simulink model "channelizer_FIR1"  (R2025a)
settings: Solver=VariableStepAuto  StartTime=0.0  StopTime=4000/100e6  RelTol=1e-3
InitFcn:
  | num_chan = 8;  % Number of channels
  | taps_per_phase = 20; % Number of taps per channel.
  | count = 1;
  | for i=0:1:num_chan-1 % number of channels
  |       coeffs_set_num(count:count+taps_per_phase+2) = i;
  |       count = count + taps_per_phase+2;
  |      if i == 0
  |        coeffs_set_num(count:count+5) = 0;
  |        count = count + 5;
  |      else
  |        coeffs_set_num(count:count+2) = 0;
  |        count = count + 2;
  |     end
  | 
  | end
  | 
  | coeffs_set_num = coeffs_set_num(1:160);
  | coeffs_tlast = [zeros(1,num_chan)];
  | for k=1:1:39
  | coeffs_tlast = [coeffs_tlast,1,zeros(1,(num_chan/2)-1)];
  | end
  | coeffs_tlast = coeffs_tlast(1:160);
undefined symbols (not defined in the file or in its folder): dspblkCoreblockFVToolHelper, es1, gcbh, S, vsva2488, xcvr1602
libraries: hdlBasic x30, dspsrcs4 x4, dspswit3 x2, hdlDSPIP x1, vmcUtilities x1
settings Model: Creator=nanumolu  LastModifiedBy=sdegala

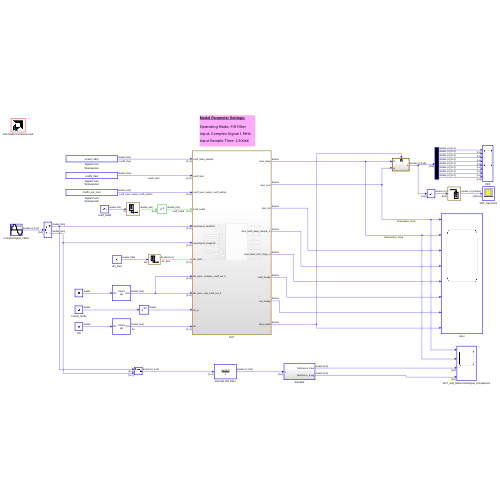
[thumbnail: Simulink's stored preview of the top-level diagram]
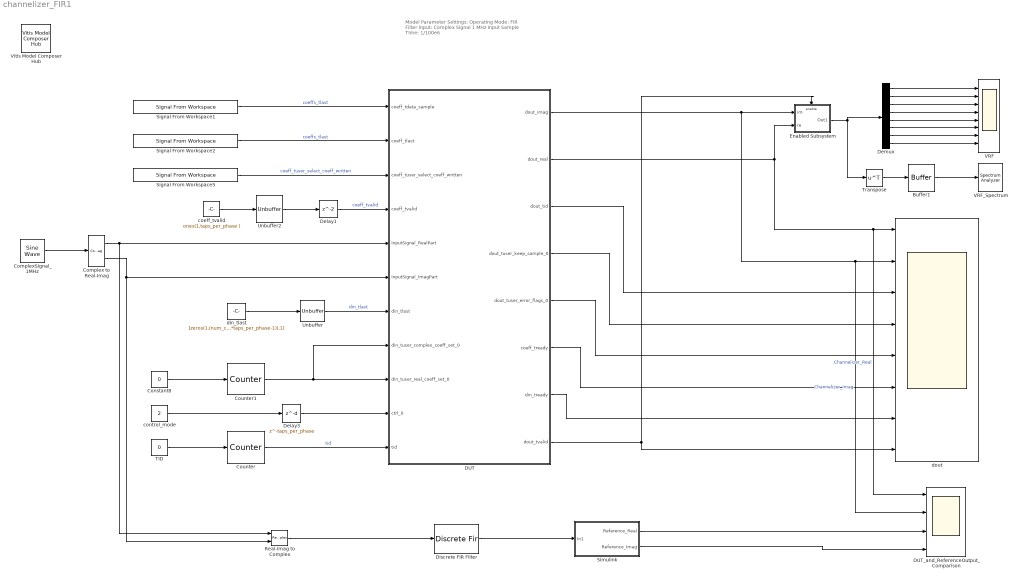
== system channelizer_FIR1 ==
  note: Model Parameter Settings:
      |
      | Operating Mode: FIR Filter
      | Input: Complex Signal 1 MHz
      | Input Sample TIme: 1/100e6
  Buffer1 : Buffer  N=1024  OutputFrames=off
  Complex to Real-Imag : ComplexToRealImag
  ComplexSignal_1MHz : dspsrcs4/Sine Wave  Amplitude=0.15  Frequency=1e6  Phase=0  SampleMode=Discrete  OutComplex=Complex  CompMethod=Trigonometric fcn  TableSize=Speed  SampleTime=1/100e6  SamplesPerFrame=1  ResetState=Restart at time zero  OutputFrames=off  dataType=double  wordLen=16  udDataType=sfix(16)  fracBitsMode=Best precision  numFracBits=15  OutDataTypeStr=double  LastOutDataTypeStr=double
  Constant8 : Constant  Value=0  SampleTime=1/100e6
  Counter : dspswit3/Counter  Direction=Up  CountEvent=Non-zero sample  CounterSize=User defined  MaxCount=num_chan-1  InitialCount=0  Output=Count  HitValue=32  ResetInput=off  SamplesPerFrame=1  Ts=1  CntDtype=double  HitDtype=Logical
  Counter1 : dspswit3/Counter  Direction=Up  CountEvent=Non-zero sample  CounterSize=User defined  MaxCount=num_chan-1  InitialCount=0  Output=Count  HitValue=32  ResetInput=off  SamplesPerFrame=1  Ts=1  CntDtype=double  HitDtype=Logical
  DUT : Subsystem
  DUT_and_ReferenceOutput_Comparison : Scope  NumInputPorts=4
      settings: ActiveDisplayYMinimum=-0.44039726257324219  ActiveDisplayYMaximum=0.44039726257324219
  Delay1 : Delay
  Delay3 : Delay  DelayLength=taps_per_phase
  Demux : Demux  Outputs=8
  Discrete FIR Filter : DiscreteFir  LoadFcn=dspblkCoreblockFVToolHelper(gcbh,'load');  Coefficients=ones(1,20)  InputProcessing=Columns as channels (frame based)  OutDataTypeStr=Inherit: Same as input
      settings: CopyFcn=dspblkCoreblockFVToolHelper(gcbh,'copy');  DeleteFcn=dspblkCoreblockFVToolHelper(gcbh,'close');  ModelCloseFcn=dspblkCoreblockFVToolHelper(gcbh,'close');  PreSaveFcn=dspblkCoreblockFVToolHelper(gcbh,'presave');  PostSaveFcn=dspblkCoreblockFVToolHelper(gcbh,'postsave');  CloseFcn=dspblkCoreblockFVToolHelper(gcbh,'close');
  Enabled Subsystem : Subsystem  TreatAsAtomicUnit=on
  Real-Imag to Complex : RealImagToComplex
  Signal From Workspace1 : dspsrcs4/Signal From Workspace  X=ones(1,160)  Ts=1/100e6  nsamps=1  OutputAfterFinalValue=Setting to zero  ignoreOrWarnInputAndFrameLengths=off  OutputFrames=off
  Signal From Workspace2 : dspsrcs4/Signal From Workspace  X=coeffs_tlast  Ts=1/100e6  nsamps=1  OutputAfterFinalValue=Setting to zero  ignoreOrWarnInputAndFrameLengths=off  OutputFrames=off
  Signal From Workspace5 : dspsrcs4/Signal From Workspace  X=coeffs_set_num  Ts=1/100e6  nsamps=1  OutputAfterFinalValue=Setting to zero  ignoreOrWarnInputAndFrameLengths=off  OutputFrames=off
  Simulink : Subsystem
  TID : Constant  Value=0  SampleTime=1
  Transpose : Math  Operator=transpose
  Unbuffer : Unbuffer
  Unbuffer2 : Unbuffer
  VRF : Scope  NumInputPorts=8
      settings: TimeUnits=Metric (based on Time Span)  ActiveDisplayYMinimum=-0.43884372711181641  ActiveDisplayYMaximum=0.44022464752197266  YLabel=Amplitude  DataLoggingVariableName=ScopeData3
  VRF_Spectrum : SpectrumAnalyzer  WindowPosition=[1.000000,1.000000,1920.000000,1127.000000,]  Visible=on  ScopeFrameLocation=window  WindowInvariantSamplesPerUpdate=on  Span=100000000  StartFrequency=-50000000  StopFrequency=50000000  YLimits=[-3603.4449 -2802.6794]
  Vitis Model Composer Hub : vmcUtilities/Vitis Model Composer Hub  Tag=genX  CodeGeneration=off  SubsystemName=DUT  BlockHierPath=Channalizer_smoke  CompilationType=HDLCompilation  SubsystemType=HDLNode  ExportTypeV2=HDL Netlist  StartColumn=1  NumberOfColumns=1  TargetDirectory=./netlist_chan_vlg  exportDesign=on  analyzeDesign=off  validateDesignOnHw=off  ExportType=AI Engines  IpVendor=xilinx.com  IpLibrary=hls  IpVersion=1.0  IpHWLanguage=Verilog  AieCompilerOptions={}  AieSimulatorOptions={}  CreateTestbench=on  TestbenchStackSize=10  RunRtlSim=off  RunCSim=off  RunAieSim=off  AieSimTimeout=50000  RunAieSimProfiling=off  LaunchVitisAnalyzer=off  PlotOutput=off  RunX86Sim=off  X86SimTimeout=10  GenHwImage=off  GenLibadfXo=on  GenHwValidationCode=off  PlatformType=Not Specified  HwSystemType=Baremetal  HwValidationTarget=hw  ProjDevice=xcvr1602-vsva2488-2MP-e-S-es1  ProjDevicePart=xcvr1602-vsva2488-2MP-e-S-es1  AIEType=AIE  SamplePeriod=-1  ClockFrequency=200  DataPathParallelism=1  xilinxfamily=versalairfes1  part=xcvr1602  speed=-2MP-e-S-es1  package=vsva2488  directory=./netlist/ip/DUT/src  testbench=off  incr_netlist=off  synthesis_tool=Vivado  clock_wrapper=Clock Enables  dbl_ovrd=According to Block Masks  dcm_input_clock_period=10  sysclk_period=10  simulink_period=1/100e6  eval_field=0  IPInfoJsonString="{\"DUTSubsystemName\":\"Channalizer_smoke\",\"HDLSubsystem\":{\"SubsystemName\":\"Channalizer_smoke\",\"IPName\":\"Copy_of_hamilton_vrf_fft\",\"IPLibrary\":\"VMC\",\"IPVendor\":\"User Company\",\"IPVersion\":\"1.0\",\"TargetDirectory\":\"./netlist_chan_vlg\",\"SubsystemDir\":\"./netlist_chan_vlg/ip/Channalizer_smoke\",\"FreqHz\":\"100000000\"},\"SubsystemTag\":\"HDLNode\"}"  LogFileName=/proj/dsv_xhd/ravalib/Head/Tests/REL/2025.1/dsv/modelcomposer/hdl/regression/channelizer/smoke/netlist_chan_vlg/model_composer.log  NThreads=4  IPConfigFile=/tmp/vmctmp-10364637636032824832/Channalizer_smoke_ipconfig.json
  coeff_tvalid : Constant  Value=ones(1,taps_per_phase )  SampleTime=1/100e6
  control_mode : Constant  Value=2  SampleTime=1/100e6
  din_tlast : Constant  Value=[zeros(1,(num_chan*taps_per_phase-1)),1]  SampleTime=1/100e6
  dout : Scope  NumInputPorts=8
      settings: ActiveDisplayYMinimum=-0.44039726257324219  ActiveDisplayYMaximum=0.44039726257324219
  wires:
  Delay1/1 -> DUT/4(coeff_tvalid)  "coeff_tvalid"
  Unbuffer/1 -> DUT/7(din_tlast)  "din_tlast"
  Counter1/1 -> DUT/8(din_tuser_complex_coeff_set_0), DUT/9(din_tuser_real_coeff_set_0)
  Complex to Real-Imag/2 -> Real-Imag to Complex/2, DUT/6(InputSignal_ImagPart)
  din_tlast/1 -> Unbuffer/1
  TID/1 -> Counter/1
  coeff_tvalid/1 -> Unbuffer2/1
  Unbuffer2/1 -> Delay1/1
  control_mode/1 -> Delay3/1
  Constant8/1 -> Counter1/1
  DUT/2(dout_real) -> Enabled Subsystem/2(re), DUT_and_ReferenceOutput_Comparison/1, dout/1  "Channelizer_Real"
  DUT/1(dout_imag) -> Enabled Subsystem/1(im), dout/2, DUT_and_ReferenceOutput_Comparison/2  "Channelizer_Imag"
  Signal From Workspace5/1 -> DUT/3(coeff_tuser_select_coeff_written)  "coeff_tuser_select_coeff_written"
  DUT/3(dout_tid) -> dout/3
  DUT/4(dout_tuser_keep_sample_0) -> dout/4
  DUT/5(dout_tuser_error_flags_0) -> dout/5
  DUT/6(coeff_tready) -> dout/6
  DUT/7(din_tready) -> dout/7
  Enabled Subsystem/1(Out1) -> Demux/1, Transpose/1
  Buffer1/1 -> VRF_Spectrum/1
  Signal From Workspace2/1 -> DUT/2(coeff_tlast)  "coeffs_tlast"
  Transpose/1 -> Buffer1/1
  Demux/1 -> VRF/1
  Demux/2 -> VRF/2
  Demux/3 -> VRF/3
  Demux/4 -> VRF/4
  Demux/5 -> VRF/5
  Demux/6 -> VRF/6
  Demux/7 -> VRF/7
  Demux/8 -> VRF/8
  Real-Imag to Complex/1 -> Discrete FIR Filter/1
  Delay3/1 -> DUT/10(ctrl_0)
  Counter/1 -> DUT/11(tid)  "tid"
  Complex to Real-Imag/1 -> Real-Imag to Complex/1, DUT/5(InputSignal_RealPart)
  DUT/8(dout_tvalid) -> Enabled Subsystem/Enable, dout/8
  Discrete FIR Filter/1 -> Simulink/1(In1)
  Simulink/1(Reference_Real) -> DUT_and_ReferenceOutput_Comparison/3
  Simulink/2(Reference_Imag) -> DUT_and_ReferenceOutput_Comparison/4
  ComplexSignal_1MHz/1 -> Complex to Real-Imag/1
  Signal From Workspace1/1 -> DUT/1(coeff_tdata_sample)  "coeffs_tlast"

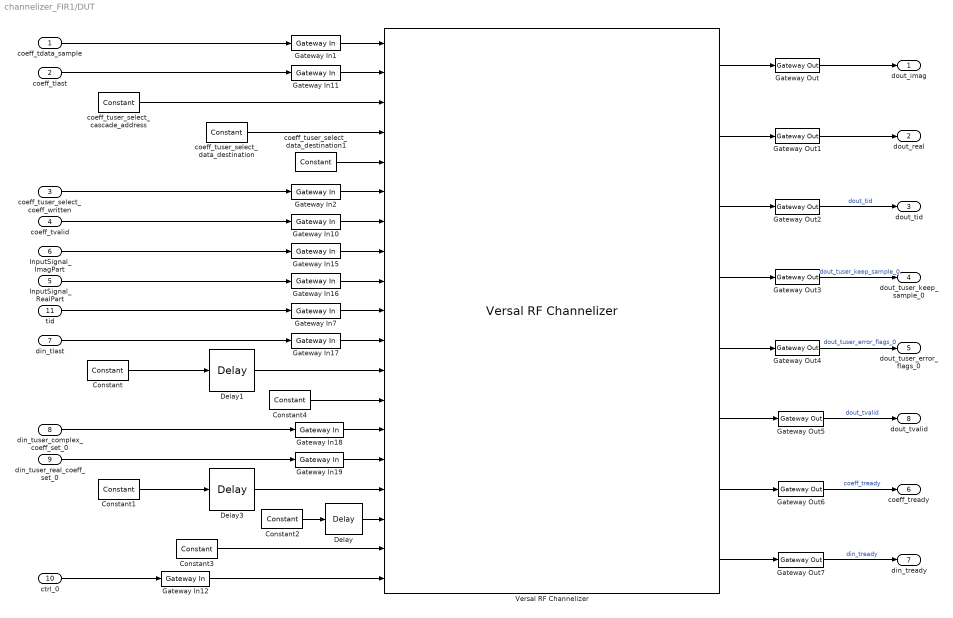
== system channelizer_FIR1/DUT ==
  coeff_tdata_sample : Inport
  coeff_tlast : Inport  Port=2
  coeff_tuser_select_coeff_written : Inport  Port=3
  coeff_tvalid : Inport  Port=4
  InputSignal_RealPart : Inport  Port=5
  InputSignal_ImagPart : Inport  Port=6
  din_tlast : Inport  Port=7
  din_tuser_complex_coeff_set_0 : Inport  Port=8
  din_tuser_real_coeff_set_0 : Inport  Port=9
  ctrl_0 : Inport  Port=10
  tid : Inport  Port=11
  Constant : hdlBasic/Constant  const=1.0  gui_display_data_type=Fixed-point  arith_type=Unsigned  n_bits=1  bin_pt=0  preci_type=Single  exp_width=8  frac_width=24  explicit_period=on  period=1/100e6  XmcBlockStatus=1  maskContainerNames=tabcontainer1  block_type=constant  block_config=sysgen:Constant_config
  Constant1 : hdlBasic/Constant  const=1.0  gui_display_data_type=Boolean  arith_type=Boolean  n_bits=1  bin_pt=0  preci_type=Single  exp_width=8  frac_width=24  explicit_period=on  period=1/100e6  XmcBlockStatus=1  maskContainerNames=tabcontainer1  block_type=constant  block_config=sysgen:Constant_config
  Constant2 : hdlBasic/Constant  const=1.0  gui_display_data_type=Boolean  arith_type=Boolean  n_bits=1  bin_pt=0  preci_type=Single  exp_width=8  frac_width=24  explicit_period=on  period=1/100e6  XmcBlockStatus=1  maskContainerNames=tabcontainer1  block_type=constant  block_config=sysgen:Constant_config
  Constant3 : hdlBasic/Constant  const=1.0  gui_display_data_type=Boolean  arith_type=Boolean  n_bits=1  bin_pt=0  preci_type=Single  exp_width=8  frac_width=24  explicit_period=on  period=1/100e6  XmcBlockStatus=1  maskContainerNames=tabcontainer1  block_type=constant  block_config=sysgen:Constant_config
  Constant4 : hdlBasic/Constant  const=1.0  gui_display_data_type=Fixed-point  arith_type=Unsigned  n_bits=1  bin_pt=0  preci_type=Single  exp_width=8  frac_width=24  explicit_period=on  period=1/100e6  XmcBlockStatus=1  maskContainerNames=tabcontainer1  block_type=constant  block_config=sysgen:Constant_config
  Delay : hdlBasic/Delay  rst=off  en=off  latency=2  reg_retiming=off  XmcBlockStatus=1  maskContainerNames=group1  block_type=delay  block_config=sysgen:Delay_config
  Delay1 : hdlBasic/Delay  rst=off  en=off  latency=num_chan*taps_per_phase  reg_retiming=off  XmcBlockStatus=1  maskContainerNames=group1  block_type=delay  block_config=sysgen:Delay_config
  Delay3 : hdlBasic/Delay  rst=off  en=off  latency=num_chan*taps_per_phase  reg_retiming=off  XmcBlockStatus=1  maskContainerNames=group1  block_type=delay  block_config=sysgen:Delay_config
  Gateway In1 : hdlBasic/Gateway In  gui_display_data_type=Fixed-point  arith_type=Signed (2's comp)  n_bits=18  bin_pt=17  preci_type=Single  exp_width=8  frac_width=24  rows=1  columns=1  quantization="Round  (unbiased: +/- Inf)"  overflow=Saturate  period=1/100e6  UseAsADC=off  ADCChannel='1'  interface=None  automatic_assignment=on  address_offset=hex2dec('00')  intf_name=''  intf_description=''  default_value=0  timing_constraint=None  locs_specified=off  LOCs={}  io_standard={}  inherit_from_input=off  hdl_port=on  XmcBlockStatus=1  maskContainerNames=group4  block_type=gatewayin  block_config=sysgen:gateway_in_config  block_width_w=590  block_height_w=620  block_width=640  block_height=850
  Gateway In10 : hdlBasic/Gateway In  gui_display_data_type=Boolean  arith_type=Boolean  n_bits=16  bin_pt=14  preci_type=Single  exp_width=8  frac_width=24  rows=1  columns=1  quantization="Round  (unbiased: +/- Inf)"  overflow=Saturate  period=1/100e6  UseAsADC=off  ADCChannel='1'  interface=None  automatic_assignment=on  address_offset=hex2dec('00')  intf_name=''  intf_description=''  default_value=0  timing_constraint=None  locs_specified=off  LOCs={}  io_standard={}  inherit_from_input=off  hdl_port=on  XmcBlockStatus=1  maskContainerNames=group4  block_type=gatewayin  block_config=sysgen:gateway_in_config  block_width_w=590  block_height_w=620  block_width=640  block_height=850
  Gateway In11 : hdlBasic/Gateway In  gui_display_data_type=Boolean  arith_type=Boolean  n_bits=16  bin_pt=14  preci_type=Single  exp_width=8  frac_width=24  rows=1  columns=1  quantization="Round  (unbiased: +/- Inf)"  overflow=Saturate  period=1/100e6  UseAsADC=off  ADCChannel='1'  interface=None  automatic_assignment=on  address_offset=hex2dec('00')  intf_name=''  intf_description=''  default_value=0  timing_constraint=None  locs_specified=off  LOCs={}  io_standard={}  inherit_from_input=off  hdl_port=on  XmcBlockStatus=1  maskContainerNames=group4  block_type=gatewayin  block_config=sysgen:gateway_in_config  block_width_w=590  block_height_w=620  block_width=640  block_height=850
  Gateway In12 : hdlBasic/Gateway In  gui_display_data_type=Fixed-point  arith_type=Signed (2's comp)  n_bits=8  bin_pt=0  preci_type=Single  exp_width=8  frac_width=24  rows=1  columns=1  quantization="Round  (unbiased: +/- Inf)"  overflow=Saturate  period=1/100e6  UseAsADC=off  ADCChannel='1'  interface=None  automatic_assignment=on  address_offset=hex2dec('00')  intf_name=''  intf_description=''  default_value=0  timing_constraint=None  locs_specified=off  LOCs={}  io_standard={}  inherit_from_input=off  hdl_port=on  XmcBlockStatus=1  maskContainerNames=group4  block_type=gatewayin  block_config=sysgen:gateway_in_config  block_width_w=590  block_height_w=620  block_width=640  block_height=850
  Gateway In15 : hdlBasic/Gateway In  gui_display_data_type=Fixed-point  arith_type=Signed (2's comp)  n_bits=18  bin_pt=17  preci_type=Single  exp_width=8  frac_width=24  rows=1  columns=1  quantization="Round  (unbiased: +/- Inf)"  overflow=Saturate  period=1/100e6  UseAsADC=off  ADCChannel='1'  interface=None  automatic_assignment=on  address_offset=hex2dec('00')  intf_name=''  intf_description=''  default_value=0  timing_constraint=None  locs_specified=off  LOCs={}  io_standard={}  inherit_from_input=off  hdl_port=on  XmcBlockStatus=1  maskContainerNames=group4  block_type=gatewayin  block_config=sysgen:gateway_in_config  block_width_w=590  block_height_w=620  block_width=640  block_height=850
  Gateway In16 : hdlBasic/Gateway In  gui_display_data_type=Fixed-point  arith_type=Signed (2's comp)  n_bits=18  bin_pt=17  preci_type=Single  exp_width=8  frac_width=24  rows=1  columns=1  quantization="Round  (unbiased: +/- Inf)"  overflow=Saturate  period=1/100e6  UseAsADC=off  ADCChannel='1'  interface=None  automatic_assignment=on  address_offset=hex2dec('00')  intf_name=''  intf_description=''  default_value=0  timing_constraint=None  locs_specified=off  LOCs={}  io_standard={}  inherit_from_input=off  hdl_port=on  XmcBlockStatus=1  maskContainerNames=group4  block_type=gatewayin  block_config=sysgen:gateway_in_config  block_width_w=590  block_height_w=620  block_width=640  block_height=850
  Gateway In17 : hdlBasic/Gateway In  gui_display_data_type=Boolean  arith_type=Boolean  n_bits=16  bin_pt=14  preci_type=Single  exp_width=8  frac_width=24  rows=1  columns=1  quantization="Round  (unbiased: +/- Inf)"  overflow=Saturate  period=1/100e6  UseAsADC=off  ADCChannel='1'  interface=None  automatic_assignment=on  address_offset=hex2dec('00')  intf_name=''  intf_description=''  default_value=0  timing_constraint=None  locs_specified=off  LOCs={}  io_standard={}  inherit_from_input=off  hdl_port=on  XmcBlockStatus=1  maskContainerNames=group4  block_type=gatewayin  block_config=sysgen:gateway_in_config  block_width_w=590  block_height_w=620  block_width=640  block_height=850
  Gateway In18 : hdlBasic/Gateway In  gui_display_data_type=Fixed-point  arith_type=Unsigned  n_bits=3  bin_pt=0  preci_type=Single  exp_width=8  frac_width=24  rows=1  columns=1  quantization="Round  (unbiased: +/- Inf)"  overflow=Saturate  period=1/100e6  UseAsADC=off  ADCChannel='1'  interface=None  automatic_assignment=on  address_offset=hex2dec('00')  intf_name=''  intf_description=''  default_value=0  timing_constraint=None  locs_specified=off  LOCs={}  io_standard={}  inherit_from_input=off  hdl_port=on  XmcBlockStatus=1  maskContainerNames=group4  block_type=gatewayin  block_config=sysgen:gateway_in_config  block_width_w=590  block_height_w=620  block_width=640  block_height=850
  Gateway In19 : hdlBasic/Gateway In  gui_display_data_type=Fixed-point  arith_type=Unsigned  n_bits=3  bin_pt=0  preci_type=Single  exp_width=8  frac_width=24  rows=1  columns=1  quantization="Round  (unbiased: +/- Inf)"  overflow=Saturate  period=1/100e6  UseAsADC=off  ADCChannel='1'  interface=None  automatic_assignment=on  address_offset=hex2dec('00')  intf_name=''  intf_description=''  default_value=0  timing_constraint=None  locs_specified=off  LOCs={}  io_standard={}  inherit_from_input=off  hdl_port=on  XmcBlockStatus=1  maskContainerNames=group4  block_type=gatewayin  block_config=sysgen:gateway_in_config  block_width_w=590  block_height_w=620  block_width=640  block_height=850
  Gateway In2 : hdlBasic/Gateway In  gui_display_data_type=Fixed-point  arith_type=Unsigned  n_bits=3  bin_pt=0  preci_type=Single  exp_width=8  frac_width=24  rows=1  columns=1  quantization="Round  (unbiased: +/- Inf)"  overflow=Saturate  period=1/100e6  UseAsADC=off  ADCChannel='1'  interface=None  automatic_assignment=on  address_offset=hex2dec('00')  intf_name=''  intf_description=''  default_value=0  timing_constraint=None  locs_specified=off  LOCs={}  io_standard={}  inherit_from_input=off  hdl_port=on  XmcBlockStatus=1  maskContainerNames=group4  block_type=gatewayin  block_config=sysgen:gateway_in_config  block_width_w=590  block_height_w=620  block_width=640  block_height=850
  Gateway In7 : hdlBasic/Gateway In  gui_display_data_type=Fixed-point  arith_type=Signed (2's comp)  n_bits=3  bin_pt=0  preci_type=Single  exp_width=8  frac_width=24  rows=1  columns=1  quantization="Round  (unbiased: +/- Inf)"  overflow=Saturate  period=1/100e6  UseAsADC=off  ADCChannel='1'  interface=None  automatic_assignment=on  address_offset=hex2dec('00')  intf_name=''  intf_description=''  default_value=0  timing_constraint=None  locs_specified=off  LOCs={}  io_standard={}  inherit_from_input=off  hdl_port=on  XmcBlockStatus=1  maskContainerNames=group4  block_type=gatewayin  block_config=sysgen:gateway_in_config  block_width_w=590  block_height_w=620  block_width=640  block_height=850
  Gateway Out{,1..7} (8 alike) : hdlBasic/Gateway Out  inherit_from_input=off  bool_to_boolean=off  hdl_port=on  rows=1  columns=1  UseAsDAC=off  DACChannel='1'  interface=None  automatic_assignment=on  address_offset=hex2dec('00')  intf_name=''  intf_description=''  timing_constraint=None  locs_specified=off  LOCs={}  io_standard={}  XmcBlockStatus=1  maskContainerNames=group4  block_type=gatewayout  block_config=sysgen:gateway_out_config  block_width_w=590  block_height_w=620  block_width=620  block_height=750
  Versal RF Channelizer : hdlDSPIP/Versal RF Channelizer  mode=FIR Filter  input_sample_rate=1  num_of_instances=1  fft_direction=FFT  fft_sync_on_tlast=off  fir_coeff_type=Real  fir_length=16  gain_en=off  events=off  coeff_casc_en=off  active_duty_cycle=25  toggle_rate=25  fir_unit_0_taps=16  fir_unit_1_taps=0  fir_unit_2_taps=0  fir_unit_3_taps=0  ip_name=Versal RF Channelizer  enable_all_ports=false  ip_version=1.1  dsptool_ready=false  ipcore_usecache=true  ipcore_useipmodelcache=true  wrapper_available=true  port_translation_map={ 'aclken' => 'en', 'aresetn' => 'rst' }  structural_sim=true  ipcore_do_not_force_period=true  oldconvolution_code_radix=Binary  XmcBlockStatus=1  maskContainerNames=tabcontainer1  block_type=vrf_channelizer_v1_1  block_config=sysgen:rodinimport_config
  coeff_tuser_select_cascade_address : hdlBasic/Constant  const=0  gui_display_data_type=Fixed-point  arith_type=Unsigned  n_bits=4  bin_pt=0  preci_type=Single  exp_width=8  frac_width=24  explicit_period=on  period=1/100e6  XmcBlockStatus=1  maskContainerNames=tabcontainer1  block_type=constant  block_config=sysgen:Constant_config
  coeff_tuser_select_data_destination : hdlBasic/Constant  const=1.0  gui_display_data_type=Fixed-point  arith_type=Unsigned  n_bits=2  bin_pt=0  preci_type=Single  exp_width=8  frac_width=24  explicit_period=on  period=1/100e6  XmcBlockStatus=1  maskContainerNames=tabcontainer1  block_type=constant  block_config=sysgen:Constant_config
  coeff_tuser_select_data_destination1 : hdlBasic/Constant  const=0  gui_display_data_type=Fixed-point  arith_type=Unsigned  n_bits=1  bin_pt=0  preci_type=Single  exp_width=8  frac_width=24  explicit_period=on  period=1/100e6  XmcBlockStatus=1  maskContainerNames=tabcontainer1  block_type=constant  block_config=sysgen:Constant_config
  dout_imag : Outport
  dout_real : Outport  Port=2
  dout_tid : Outport  Port=3
  dout_tuser_keep_sample_0 : Outport  Port=4
  dout_tuser_error_flags_0 : Outport  Port=5
  coeff_tready : Outport  Port=6
  din_tready : Outport  Port=7
  dout_tvalid : Outport  Port=8
  wires:
  Gateway In11/1 -> Versal RF Channelizer/2
  coeff_tuser_select_coeff_written/1 -> Gateway In2/1
  Gateway In15/1 -> Versal RF Channelizer/8
  Versal RF Channelizer/4 -> Gateway Out3/1
  Versal RF Channelizer/6 -> Gateway Out5/1
  din_tuser_complex_coeff_set_0/1 -> Gateway In18/1
  Versal RF Channelizer/1 -> Gateway Out/1
  Constant3/1 -> Versal RF Channelizer/18
  Versal RF Channelizer/8 -> Gateway Out7/1
  Gateway Out2/1 -> dout_tid/1  "dout_tid"
  Gateway In19/1 -> Versal RF Channelizer/15
  Gateway In1/1 -> Versal RF Channelizer/1
  Versal RF Channelizer/7 -> Gateway Out6/1
  Gateway Out1/1 -> dout_real/1
  InputSignal_ImagPart/1 -> Gateway In15/1
  Gateway In12/1 -> Versal RF Channelizer/19
  coeff_tlast/1 -> Gateway In11/1
  Constant2/1 -> Delay/1
  ctrl_0/1 -> Gateway In12/1
  Gateway In18/1 -> Versal RF Channelizer/14
  din_tuser_real_coeff_set_0/1 -> Gateway In19/1
  InputSignal_RealPart/1 -> Gateway In16/1
  Gateway In2/1 -> Versal RF Channelizer/6
  Versal RF Channelizer/3 -> Gateway Out2/1
  Versal RF Channelizer/2 -> Gateway Out1/1
  coeff_tvalid/1 -> Gateway In10/1
  Delay3/1 -> Versal RF Channelizer/16
  Gateway Out7/1 -> din_tready/1  "din_tready"
  Constant4/1 -> Versal RF Channelizer/13
  din_tlast/1 -> Gateway In17/1
  Gateway Out5/1 -> dout_tvalid/1  "dout_tvalid"
  Gateway Out/1 -> dout_imag/1
  Versal RF Channelizer/5 -> Gateway Out4/1
  Gateway In16/1 -> Versal RF Channelizer/9
  Gateway In17/1 -> Versal RF Channelizer/11
  Gateway Out3/1 -> dout_tuser_keep_sample_0/1  "dout_tuser_keep_sample_0"
  Gateway Out6/1 -> coeff_tready/1  "coeff_tready"
  Gateway Out4/1 -> dout_tuser_error_flags_0/1  "dout_tuser_error_flags_0"
  Gateway In10/1 -> Versal RF Channelizer/7
  coeff_tuser_select_data_destination1/1 -> Versal RF Channelizer/5
  tid/1 -> Gateway In7/1
  Gateway In7/1 -> Versal RF Channelizer/10
  coeff_tdata_sample/1 -> Gateway In1/1
  coeff_tuser_select_cascade_address/1 -> Versal RF Channelizer/3
  coeff_tuser_select_data_destination/1 -> Versal RF Channelizer/4
  Constant/1 -> Delay1/1
  Delay1/1 -> Versal RF Channelizer/12
  Constant1/1 -> Delay3/1
  Delay/1 -> Versal RF Channelizer/17

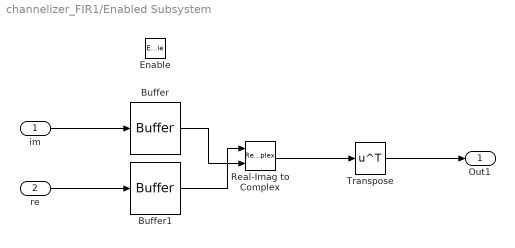
== system channelizer_FIR1/Enabled Subsystem ==
  im : Inport
  re : Inport  Port=2
  Enable : EnablePort
  Buffer : Buffer  N=num_chan  OutputFrames=off
  Buffer1 : Buffer  N=num_chan  OutputFrames=off
  Real-Imag to Complex : RealImagToComplex
  Transpose : Math  Operator=transpose
  Out1 : Outport
  wires:
  re/1 -> Buffer1/1
  im/1 -> Buffer/1
  Buffer/1 -> Real-Imag to Complex/2
  Buffer1/1 -> Real-Imag to Complex/1
  Real-Imag to Complex/1 -> Transpose/1
  Transpose/1 -> Out1/1

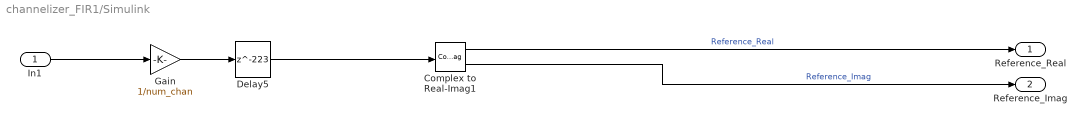
== system channelizer_FIR1/Simulink ==
  In1 : Inport
  Complex to Real-Imag1 : ComplexToRealImag
  Delay5 : Delay  DelayLength=223  DelayLengthUpperLimit=1000
  Gain : Gain  Gain=1/num_chan
  Reference_Real : Outport
  Reference_Imag : Outport  Port=2
  wires:
  Gain/1 -> Delay5/1
  Delay5/1 -> Complex to Real-Imag1/1
  Complex to Real-Imag1/1 -> Reference_Real/1  "Reference_Real"
  Complex to Real-Imag1/2 -> Reference_Imag/1  "Reference_Imag"
  In1/1 -> Gain/1
